simulink model "dynamic_sim"  (R2016a)
settings: Solver=VariableStepAuto  StartTime=0.0  StopTime=2  FixedStep=1e-6  RelTol=1e-3
values from neighbouring files (symbols this model uses):
  F = 1e-7    (= 1e-07)    [dynamic_sim_constants.m]
  J = 1e-9    (= 1e-09)    [dynamic_sim_constants.m]
  Ki_d = 0.00001    (= 1e-05)    [dynamic_sim_constants.m]
  Ki_q = 0.00001    (= 1e-05)    [dynamic_sim_constants.m]
  Km = .00149    (= 0.00149)    [dynamic_sim_constants.m]
  Kp_d = 10    [dynamic_sim_constants.m]
  Kp_q = 10    [dynamic_sim_constants.m]
  L = 0.00001462*3/2    (= 2.193e-05)    [dynamic_sim_constants.m]    (also in serial_bin_log.m = length(log))
  P = 2    [dynamic_sim_constants.m]    (also in foc_matlab_plot.m = mean(avg_st); serial_bin_log.m = mean(avg_st); slow_1hz_current_data_2_1A.mat = 0.00101490868431; slow_1hz_current_datas.mat = 0.00101490868431)
  psi = 0.00152788745    [dynamic_sim_constants.m]
  R = .86*3/2    (= 1.29)    [dynamic_sim_constants.m]
settings Model: Creator=Ocanath  LastModifiedBy=Ocanath

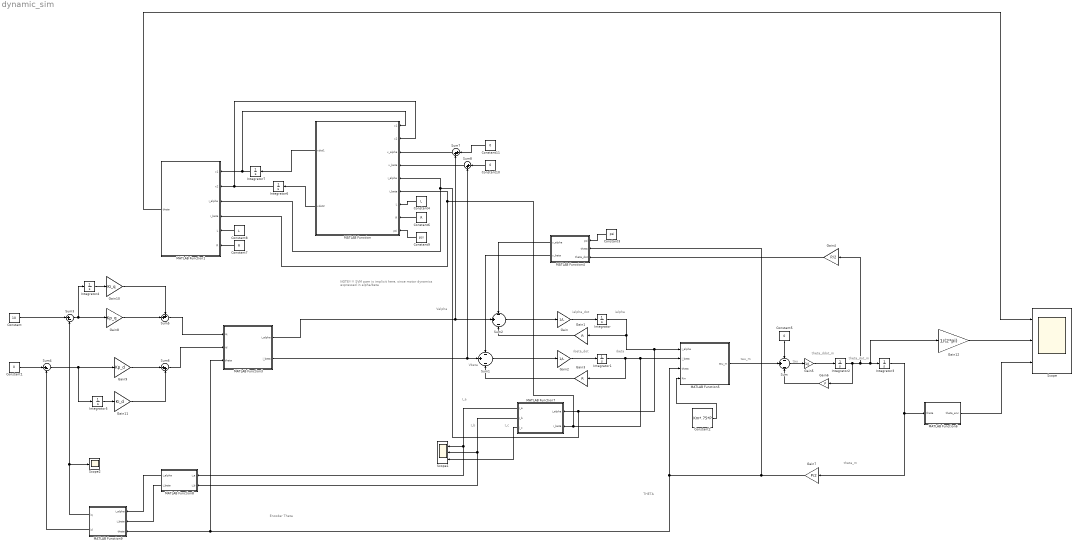
== system dynamic_sim ==
  note: THETA
  note: I_c
  note: I_b
  note: I_a
  note: Encoder Theta
  note: tau
  note: tau_m
  note: theta_ddot_m
  note: theta_dot_m
  note: theta_m
  note: ibeta
  note: ialpha
  note: ibeta_dot
  note: ialpha_dot
  note: Vbeta
  note: Valpha
  note: NOTE!!!!
      | SVM pwm is implicit here,
      | since motor dynamics expressed in
      | alpha/beta
  Constant : Constant  Value=10
  Constant{1,5,10..11} (4 alike) : Constant  Value=0
  Constant2 : Constant  Value=Km*.75*P
  Constant3 : Constant  Value=psi
  Constant4 : Constant  Value=L
  Constant6 : Constant  Value=R
  Constant7 : Constant  Value=R
  Constant8 : Constant  Value=L
  Constant9 : Constant  Value=psi
  Gain : Gain  Gain=1/L
  Gain1 : Gain  Gain=R
  Gain10 : Gain  Gain=Ki_q
  Gain11 : Gain  Gain=Ki_d
  Gain12 : Gain  Gain=1/(2*pi)
  Gain2 : Gain  Gain=1/L
  Gain3 : Gain  Gain=R
  Gain4 : Gain  Gain=P/2
  Gain5 : Gain  Gain=1/J
  Gain6 : Gain  Gain=F
  Gain7 : Gain  Gain=P/2
  Gain8 : Gain  Gain=Kp_q
  Gain9 : Gain  Gain=Kp_d
  Integrator{,1..7} (8 alike) : Integrator
  MATLAB Function : MATLAB Function  TreatAsAtomicUnit=on
  MATLAB Function1 : MATLAB Function  TreatAsAtomicUnit=on
  MATLAB Function3 : MATLAB Function  TreatAsAtomicUnit=on
  MATLAB Function4 : MATLAB Function  TreatAsAtomicUnit=on
  MATLAB Function5 : MATLAB Function  TreatAsAtomicUnit=on
  MATLAB Function6 : MATLAB Function  TreatAsAtomicUnit=on
  MATLAB Function7 : MATLAB Function  TreatAsAtomicUnit=on
  MATLAB Function8 : MATLAB Function  TreatAsAtomicUnit=on
  MATLAB Function9 : MATLAB Function  TreatAsAtomicUnit=on
  Scope : Scope  NumInputPorts=3
  Scope1 : Scope  NumInputPorts=3
  Scope2 : Scope
  Sum : Sum  Inputs=-|+|-
  Sum1 : Sum  Inputs=-|+|-
  Sum2 : Sum  Inputs=-|+|-
  Sum3 : Sum  Inputs=|+-
  Sum4 : Sum  Inputs=|+-
  Sum5 : Sum  Inputs=++|
  Sum6 : Sum  Inputs=|++
  Sum7 : Sum  Inputs=|++
  Sum8 : Sum  Inputs=|++
  wires:
  Sum2/1 -> Gain/1
  Gain/1 -> Integrator/1
  Gain1/1 -> Sum2/3
  MATLAB Function3/1(i_alpha) -> Sum2/2, Sum7/2
  Sum1/1 -> Gain2/1
  Gain2/1 -> Integrator1/1
  Gain3/1 -> Sum1/3
  MATLAB Function4/1(v_alpha) -> Sum2/1
  MATLAB Function4/2(v_beta) -> Sum1/1
  Constant2/1 -> MATLAB Function5/4(Km)
  MATLAB Function5/1(tau_m) -> Sum/2
  Constant5/1 -> Sum/1
  Sum/1 -> Gain5/1
  Gain6/1 -> Sum/3
  Integrator3/1 -> Gain7/1, MATLAB Function6/1(theta)
  Integrator2/1 -> Gain4/1, Integrator3/1, Gain12/1, Gain6/1
  Gain5/1 -> Integrator2/1
  MATLAB Function7/1(i_a) -> Scope1/1, MATLAB Function8/1(i_a)
  MATLAB Function7/2(i_b) -> Scope1/2, MATLAB Function8/2(i_b)
  MATLAB Function8/2(i_beta) -> MATLAB Function9/2(i_beta)
  MATLAB Function8/1(i_alpha) -> MATLAB Function9/1(i_alpha)
  MATLAB Function9/1(iq) -> Scope2/1, Sum3/2
  MATLAB Function9/2(id) -> Sum4/2
  Sum3/1 -> Gain8/1, Integrator4/1
  Constant/1 -> Sum3/1
  Constant1/1 -> Sum4/1
  Sum4/1 -> Integrator5/1, Gain9/1
  Integrator4/1 -> Gain10/1
  Integrator5/1 -> Gain11/1
  Gain8/1 -> Sum5/2
  Gain10/1 -> Sum5/1
  Gain9/1 -> Sum6/1
  Gain11/1 -> Sum6/2
  Constant3/1 -> MATLAB Function4/1(psi)
  MATLAB Function6/1(theta_enc) -> Scope/3
  Gain4/1 -> MATLAB Function4/3(theta_dot)
  MATLAB Function7/3(i_c) -> Scope1/3
  Gain12/1 -> Scope/2
  Sum5/1 -> MATLAB Function3/1(iq)
  Sum6/1 -> MATLAB Function3/2(id)
  Gain7/1 -> MATLAB Function5/3(theta), MATLAB Function3/3(theta), MATLAB Function9/3(theta), MATLAB Function4/2(theta)
  MATLAB Function/2(xdot2) -> Integrator6/1
  MATLAB Function/1(xdot1) -> Integrator7/1
  Integrator1/1 -> Gain3/1, MATLAB Function1/4(i_beta), MATLAB Function/6(i_beta), MATLAB Function7/2(i_beta), MATLAB Function5/2(i_beta)
  Integrator/1 -> MATLAB Function/5(i_alpha), MATLAB Function1/3(i_alpha), MATLAB Function7/1(i_alpha), MATLAB Function5/1(i_alpha), Gain1/1
  Sum7/1 -> MATLAB Function/3(v_alpha)
  Sum8/1 -> MATLAB Function/4(v_beta)
  MATLAB Function3/2(i_beta) -> Sum1/2, Sum8/2
  MATLAB Function1/1(theta) -> Scope/1
  Constant4/1 -> MATLAB Function/7(L)
  Constant6/1 -> MATLAB Function/8(R)
  Constant7/1 -> MATLAB Function1/6(R)
  Constant8/1 -> MATLAB Function1/5(L)
  Integrator7/1 -> MATLAB Function/1(x1), MATLAB Function1/1(x1)
  Integrator6/1 -> MATLAB Function/2(x2), MATLAB Function1/2(x2)
  Constant9/1 -> MATLAB Function/9(psi)
  Constant10/1 -> Sum8/1
  Constant11/1 -> Sum7/1

== matlab function dynamic_sim/MATLAB Function1 ==
  data: x1 input; theta output; x2 input; i_alpha input; i_beta input; L input; R input
function theta = position_estimator(x1, x2, i_alpha, i_beta, L, R)
theta = atan2((x2 - L*i_beta),-(x1-L*i_alpha));
end

== matlab function dynamic_sim/MATLAB Function ==
  data: x1 input; x2 input; v_alpha input; xdot1 output; v_beta input; i_alpha input; i_beta input; xdot2 output; L input; R input; psi input
function [xdot1,xdot2] = observer( x1, x2, v_alpha,v_beta,i_alpha,i_beta, L, R, psi)
    y1 = -R*i_alpha + v_alpha;
    y2 = -R*i_beta + v_beta;
    
    n1 = x1 - L*i_alpha;
    n2 = x2 - L*i_beta;
    
    gamma = 1000;
    scale = (psi*psi- (n1*n1+n2*n2));
    xdot1 = y1 + gamma * n1 * scale;
    xdot2 = y2 + gamma * n2 * scale; 
end

== matlab function dynamic_sim/MATLAB Function3 ==
  data: iq input; i_alpha output; id input; theta input; i_beta output
function [i_alpha,i_beta] = inverse_park(iq, id, theta)
    sin_theta = sin(theta);
    cos_theta = cos(theta);
    i_alpha = id*cos_theta - iq*sin_theta;
	i_beta = id*sin_theta + iq*cos_theta;
end

== matlab function dynamic_sim/MATLAB Function4 ==
  data: psi input; theta input; theta_dot input; v_alpha output; v_beta output
function [v_alpha,v_beta] = bemf(psi, theta, theta_dot)
% v_alpha = theta_dot * psi * sin(theta);
% v_beta = -theta_dot * psi * cos(theta);

v_alpha = - theta_dot * psi * cos(theta);
v_beta = theta_dot * psi * sin(theta);
end

== matlab function dynamic_sim/MATLAB Function5 ==
  data: i_alpha input; tau_m output; i_beta input; theta input; Km input
function tau_m = fcn(i_alpha, i_beta, theta, Km)
%     tau_m = Km*(i_alpha * cos(theta) - i_beta*sin(theta));
tau_m = Km*(-i_alpha*sin(theta)+i_beta*cos(theta));
end

== matlab function dynamic_sim/MATLAB Function6 ==
  data: theta_enc output; theta input
function theta_enc = aligned_encoder(theta)
theta_enc = atan2(sin(theta),cos(theta));
end

== matlab function dynamic_sim/MATLAB Function7 ==
  data: i_alpha input; i_a output; i_beta input; i_b output; i_c output
function [i_a,i_b,i_c] = inverse_clarke(i_alpha,i_beta)
    sqrt_3_by_2 = sqrt(3)*.5;
	i_a = i_alpha;
	i_b = -.5*i_alpha + sqrt_3_by_2*i_beta;
	i_c = -.5*i_alpha - sqrt_3_by_2*i_beta;
end

== matlab function dynamic_sim/MATLAB Function8 ==
  data: i_a input; i_alpha output; i_b input; i_beta output
function [i_alpha, i_beta] = clarke(i_a, i_b)
    i_alpha = i_a;
	i_beta = (1/sqrt(3))*i_a + (2/sqrt(3))*i_b;
end

== matlab function dynamic_sim/MATLAB Function9 ==
  data: i_alpha input; iq output; i_beta input; theta input; id output
function [iq,id] = park(i_alpha, i_beta, theta)
    cos_theta = cos(theta);
    sin_theta = sin(theta);
	id = i_alpha*cos_theta+i_beta*sin_theta;
	iq = -i_alpha*sin_theta+i_beta*cos_theta;
end
